simulink model "Copy_of_shunt"  (R2021a)
settings: Solver=VariableStepAuto  StartTime=0.0  StopTime=10  FixedStep=1e-6  RelTol=1e-3
libraries: spsSeriesRLCBranchLib x10, spsCurrentMeasurementLib x9, spsIGBTDiodeLib x4, spsVoltageMeasurementLib x4, spsIGBTLib x3, spsSampleandHoldLib x3, spsGroundLib x2, spsPVArrayLib x1, spsDiodeLib x1, spsPWMGeneratorDCDCLib x1, spsThreePhaseProgrammableVoltageSourceLib x1, spsUniversalBridgeLib x1
settings Model: Creator=Dell  LastModifiedBy=Dell
settings SolverCC: ZeroCrossControl=DisableAll

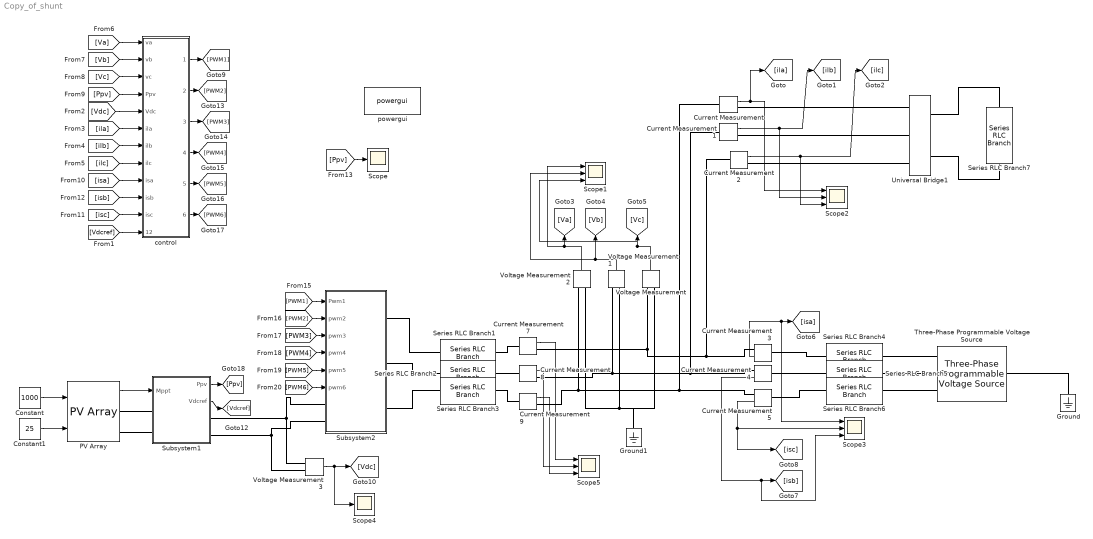
== system Copy_of_shunt ==
  Constant : Constant  Value=1000
  Constant1 : Constant  Value=25
  Current Measurement{,1..5,7..9} (9 alike) : spsCurrentMeasurementLib/Current Measurement  PhasorSimulation=off  OutputType=Complex  PSBequivalent=0
  Ground : spsGroundLib/Ground  LConnTagsString=a
  Ground1 : spsGroundLib/Ground  LConnTagsString=a
  PV Array : spsPVArrayLib/PV Array  Npar=3  Nser=25  PlotType=array @ 1000 W/m2 & specified temperatures  S_vec="[ 1000  500  100 ]"  Temp_C_vec="[ 45 25  ]"  ModuleName=User-defined  PlotWhenSelected=off  Pm=213.15  Ncell=54  Voc=36.3  Isc=7.84  Vm=29  Im=7.35  beta_Voc_pc=-0.36099  alpha_Isc_pc=0.102  beta_Voc=-0.13104  alpha_Isc=0.0079968  IL=7.8473  I0=2.9239e-10  nI=1.0901  Rsh=425.4609  Rs=0.39416  RobustModel=off  RobustCellTemperature=313.3991  BAL=on  Tc=1e-6  Tfilter=5e-5
  Scope : Scope
  Scope{1..3,5} (4 alike) : Scope  NumInputPorts=3
  Scope4 : Scope
  Series RLC Branch{1..7} (7 alike) : spsSeriesRLCBranchLib/Series RLC Branch  LConnTagsString=__new0  RConnTagsString=__new0  BranchType=RL  Resistance=1  Inductance=1e-3  SetiL0=off  InitialCurrent=0  Capacitance=1e-6  Setx0=off  InitialVoltage=0  Measurements=None
  Subsystem1 : Subsystem
  Subsystem2 : Subsystem
  Three-Phase Programmable Voltage Source : spsThreePhaseProgrammableVoltageSourceLib/Three-Phase Programmable Voltage Source  PositiveSequence="[415  0 50]"  VariationEntity=None  VariationType=Table of time-amplitude pairs  VariationTypeAlt=Step  VariationStep=0.5  VariationRate=10  VariationMagnitude=0.3  VariationFrequency=2  VariationTiming=[1 2]  VariationPhaseA=off  Amplitudes=[1 0.8 1.2 1.0]  TimeValues=[0 0.1 0.15 0.2]  HarmonicGeneration=off  HarmonicA=[3 0.2 -25 0]  HarmonicB=[2 0.15 35 2]  Timing="[0.05  3]"  BusType=swing  Pref=0  Qref=0  Qmin=-inf  Qmax=inf
  Universal Bridge1 : spsUniversalBridgeLib/Universal Bridge  Arms=3  SnubberResistance=1e5  SnubberCapacitance=inf  Device=Diodes  Ron=1e-3  Lon=0  ForwardVoltages="[  0  0  ]"  ForwardVoltage=0  GTOparameters=[ 10e-6 , 20e-6 ]  IGBTparameters=[ 1e-6 , 2e-6 ]  Measurements=None  Measurements_2=None  converterType=Rectifier
  Voltage Measurement{,1..3} (4 alike) : spsVoltageMeasurementLib/Voltage Measurement  PhasorSimulation=off  OutputType=Complex  PSBequivalent=0
  control : Subsystem
  powergui : spspowerguiLib/powergui  Priority=1  SimulationMode=Continuous  SampleTime=0.001  frequency=60  Iterations=50  frequencyindice=50  Pbase=100e6  ErrMax=1e-4  UnitsV=kV  UnitsW=MW  buscounter=0  FunctionMessages=off  echomessages=off  EnableUseOfTLC=off  CurrentSourceSwitches=off  DisableSnubberDevices=off  DisableRonSwitches=off  DisableVfSwitches=off  DisplayEquations=off  AutomaticDiscreteSolvers=off  SolverType=Tustin/Backward Euler (TBE)  Interpol=off  ExternalGateDelay=off  methode=off  Ts=100  x0status=blocks  SPID=on  SwTol=0  HookPort=off  NonlinearTolerance=1e-4  nMaxIteration=100  ContinueOnMaxIteration=off  RestoreLinks=warning  ResistiveCurrentMeasurement=off  Frange=[0:2:500]  Ylog=off  Xlog=on  ShowGrid=off  save=off  variable=ZData  structure=0  ZoomFFT=off  StartTime=0.0  cycles=1  DisplayStyle=1  fundamental=60  FreqAxis=off  MaxFrequency=1000  frequencyindicesteady=1  RmsSteady=1  display=off
  wires:
  Current Measurement/1 -> [ila], Scope2/1
  Current Measurement1/1 -> Scope2/2, [ilb]
  Current Measurement2/1 -> Scope2/3, [ilc]
  Voltage Measurement2/1 -> Scope1/1, [Va]
  Voltage Measurement1/1 -> Scope1/2, [Vb]
  Voltage Measurement/1 -> Scope1/3, [Vc]
  Current Measurement3/1 -> Scope3/1, [isa]
  Current Measurement4/1 -> Scope3/3, [isb]
  Current Measurement5/1 -> Scope3/2, [isc]
  Constant/1 -> PV Array/1
  Constant1/1 -> PV Array/2
  [Vdcref] -> control/12(Vdcref)
  [Vdc] -> control/5(Vdc)
  [ila] -> control/6(ila)
  [ilb] -> control/7(ilb)
  [ilc] -> control/8(ilc)
  [Va] -> control/1(va)
  [Vb] -> control/2(vb)
  [Vc] -> control/3(vc)
  [Ppv] -> control/4(Ppv)
  [isa] -> control/9(isa)
  [isc] -> control/11(isc)
  [isb] -> control/10(isb)
  Current Measurement7/1 -> Scope5/1
  Current Measurement8/1 -> Scope5/2
  Current Measurement9/1 -> Scope5/3
  [Ppv] -> Scope/1
  PV Array/1 -> Subsystem1/1(Mppt)
  Voltage Measurement3/1 -> Scope4/1, [Vdc]
  control/1(Output) -> [PWM1]
  control/6(Output5) -> [PWM6]
  control/5(Output4) -> [PWM5]
  control/4(Output3) -> [PWM4]
  control/3(Output2) -> [PWM3]
  control/2(Output1) -> [PWM2]
  [PWM1] -> Subsystem2/1(Pwm1)
  [PWM2] -> Subsystem2/2(pwm2)
  [PWM3] -> Subsystem2/3(pwm3)
  [PWM4] -> Subsystem2/4(pwm4)
  [PWM5] -> Subsystem2/5(pwm5)
  [PWM6] -> Subsystem2/6(pwm6)
  Subsystem1/2(Vdcref) -> [Vdcref]
  Subsystem1/1(Ppv) -> [Ppv]
  connections:
  Universal Bridge1/LConn3 -- Current Measurement/RConn1
  Universal Bridge1/LConn1 -- Current Measurement2/RConn1
  Ground/LConn1 -- Three-Phase Programmable Voltage Source/LConn1
  Current Measurement1/LConn1 -- Current Measurement8/RConn1 -- Voltage Measurement1/LConn1 -- Current Measurement4/RConn1
  Three-Phase Programmable Voltage Source/RConn1 -- Series RLC Branch4/RConn1
  Three-Phase Programmable Voltage Source/RConn2 -- Series RLC Branch5/RConn1
  Three-Phase Programmable Voltage Source/RConn3 -- Series RLC Branch6/RConn1
  Universal Bridge1/RConn1 -- Series RLC Branch7/LConn1
  Universal Bridge1/RConn2 -- Series RLC Branch7/RConn1
  Current Measurement/LConn1 -- Current Measurement9/RConn1 -- Voltage Measurement2/LConn1 -- Current Measurement5/RConn1
  Universal Bridge1/LConn2 -- Current Measurement1/RConn1
  Current Measurement2/LConn1 -- Voltage Measurement/LConn1 -- Current Measurement7/RConn1 -- Current Measurement3/RConn1
  Voltage Measurement2/LConn2 -- Voltage Measurement/LConn2 -- Ground1/LConn1 -- Voltage Measurement1/LConn2
  Series RLC Branch4/LConn1 -- Current Measurement3/LConn1
  Series RLC Branch5/LConn1 -- Current Measurement4/LConn1
  Series RLC Branch6/LConn1 -- Current Measurement5/LConn1
  Current Measurement7/LConn1 -- Series RLC Branch1/RConn1
  Current Measurement8/LConn1 -- Series RLC Branch2/RConn1
  Current Measurement9/LConn1 -- Series RLC Branch3/RConn1
  Subsystem1/LConn1 -- PV Array/RConn1
  Subsystem1/LConn2 -- PV Array/RConn2
  Subsystem1/RConn1 -- Voltage Measurement3/LConn1 -- Subsystem2/LConn1
  Subsystem1/RConn2 -- Voltage Measurement3/LConn2 -- Subsystem2/LConn2
  Series RLC Branch1/LConn1 -- Subsystem2/RConn1
  Series RLC Branch2/LConn1 -- Subsystem2/RConn2
  Series RLC Branch3/LConn1 -- Subsystem2/RConn3

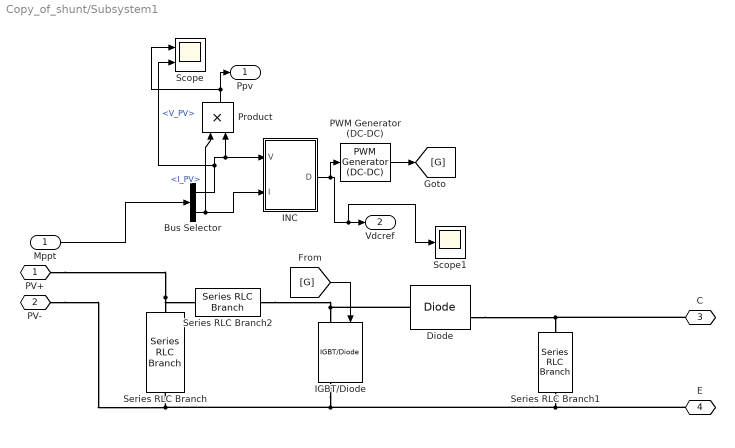
== system Copy_of_shunt/Subsystem1 ==
  Mppt : Inport
  Bus Selector : BusSelector  OutputSignals=V_PV,I_PV
  Diode : spsDiodeLib/Diode  Ron=0.001  Lon=0  Vf=0.8  IC=0  UseSnubber=0  Rs=500  Cs=250e-9  Measurements=on
  IGBT/Diode : spsIGBTDiodeLib/IGBT//Diode  Ron=1e-3  Rs=1e5  Cs=inf  Measurements=on
  INC : Subsystem
  PWM Generator (DC-DC) : spsPWMGeneratorDCDCLib/PWM Generator (DC-DC)  Fsw=5000  Ts=0
  Product : Product
  Scope : Scope  NumInputPorts=2
  Scope1 : Scope
  Series RLC Branch : spsSeriesRLCBranchLib/Series RLC Branch  LConnTagsString=__new0  RConnTagsString=__new0  BranchType=RC  Resistance=1  Inductance=1e-3  SetiL0=off  InitialCurrent=0  Capacitance=1e-6  Setx0=off  InitialVoltage=0  Measurements=None
  Series RLC Branch1 : spsSeriesRLCBranchLib/Series RLC Branch  LConnTagsString=__new0  RConnTagsString=__new0  BranchType=C  Resistance=1  Inductance=1e-3  SetiL0=off  InitialCurrent=0  Capacitance=1e-6  Setx0=off  InitialVoltage=0  Measurements=None
  Series RLC Branch2 : spsSeriesRLCBranchLib/Series RLC Branch  LConnTagsString=__new0  RConnTagsString=__new0  BranchType=L  Resistance=1  Inductance=1e-3  SetiL0=off  InitialCurrent=0  Capacitance=1e-6  Setx0=off  InitialVoltage=0  Measurements=None
  PV+ : PMIOPort  Side=Left
  PV- : PMIOPort  Port=2  Side=Left
  C : PMIOPort  Port=3  Side=Right
  E : PMIOPort  Port=4  Side=Right
  Ppv : Outport
  Vdcref : Outport  Port=2
  wires:
  INC/1(D) -> PWM Generator (DC-DC)/1, Scope1/1, Vdcref/1
  Bus Selector/2 -> INC/2(I), Product/1  "<I_PV>"
  Bus Selector/1 -> Scope/2, Product/2, INC/1(V)  "<V_PV>"
  [G] -> IGBT/Diode/1
  PWM Generator (DC-DC)/1 -> [G]
  Mppt/1 -> Bus Selector/1
  Product/1 -> Scope/1, Ppv/1
  connections:
  IGBT/Diode/RConn1 -- E/RConn1 -- Series RLC Branch1/RConn1 -- PV-/RConn1 -- Series RLC Branch/RConn1
  Diode/RConn1 -- C/RConn1 -- Series RLC Branch1/LConn1
  IGBT/Diode/LConn1 -- Series RLC Branch2/RConn1 -- Diode/LConn1
  Series RLC Branch/LConn1 -- PV+/RConn1 -- Series RLC Branch2/LConn1

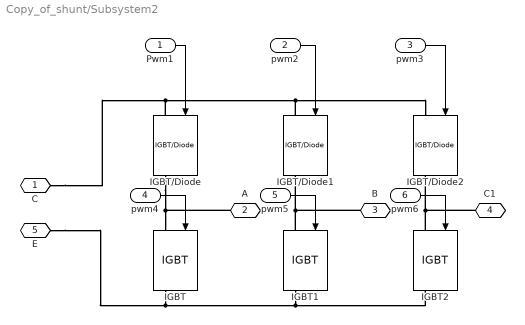
== system Copy_of_shunt/Subsystem2 ==
  Pwm1 : Inport
  pwm2 : Inport  Port=2
  pwm3 : Inport  Port=3
  pwm4 : Inport  Port=4
  pwm5 : Inport  Port=5
  pwm6 : Inport  Port=6
  IGBT : spsIGBTLib/IGBT  Ron=0.001  Lon=0  Vf=1  Tf=1e-6  Tt=2e-6  IC=0  Rs=1e5  Cs=inf  Measurements=on
  IGBT/Diode : spsIGBTDiodeLib/IGBT//Diode  Ron=1e-3  Rs=1e5  Cs=inf  Measurements=on
  IGBT/Diode1 : spsIGBTDiodeLib/IGBT//Diode  Ron=1e-3  Rs=1e5  Cs=inf  Measurements=on
  IGBT/Diode2 : spsIGBTDiodeLib/IGBT//Diode  Ron=1e-3  Rs=1e5  Cs=inf  Measurements=on
  IGBT1 : spsIGBTLib/IGBT  Ron=0.001  Lon=0  Vf=1  Tf=1e-6  Tt=2e-6  IC=0  Rs=1e5  Cs=inf  Measurements=on
  IGBT2 : spsIGBTLib/IGBT  Ron=0.001  Lon=0  Vf=1  Tf=1e-6  Tt=2e-6  IC=0  Rs=1e5  Cs=inf  Measurements=on
  C : PMIOPort  Side=Left
  A : PMIOPort  Port=2  Side=Right
  B : PMIOPort  Port=3  Side=Right
  C1 : PMIOPort  Port=4  Side=Right
  E : PMIOPort  Port=5  Side=Left
  wires:
  Pwm1/1 -> IGBT/Diode/1
  pwm6/1 -> IGBT2/1
  pwm5/1 -> IGBT1/1
  pwm4/1 -> IGBT/1
  pwm3/1 -> IGBT/Diode2/1
  pwm2/1 -> IGBT/Diode1/1
  connections:
  IGBT/Diode/RConn1 -- A/RConn1 -- IGBT/LConn1
  IGBT1/LConn1 -- B/RConn1 -- IGBT/Diode1/RConn1
  IGBT2/LConn1 -- C1/RConn1 -- IGBT/Diode2/RConn1
  IGBT/Diode/LConn1 -- C/RConn1 -- IGBT/Diode1/LConn1 -- IGBT/Diode2/LConn1
  IGBT/RConn1 -- E/RConn1 -- IGBT1/RConn1 -- IGBT2/RConn1

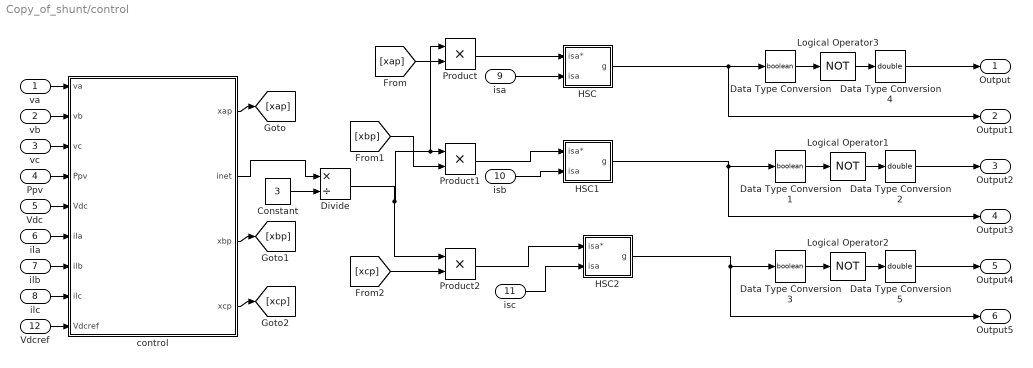
== system Copy_of_shunt/control ==
  va : Inport
  vb : Inport  Port=2
  vc : Inport  Port=3
  Ppv : Inport  Port=4
  Vdc : Inport  Port=5
  ila : Inport  Port=6
  ilb : Inport  Port=7
  ilc : Inport  Port=8
  isa : Inport  Port=9
  isb : Inport  Port=10
  isc : Inport  Port=11
  Vdcref : Inport  Port=12
  Constant : Constant  Value=3
  Data Type Conversion : DataTypeConversion  OutDataTypeStr=boolean  SaturateOnIntegerOverflow=on  RndMeth=Zero
  Data Type Conversion1 : DataTypeConversion  OutDataTypeStr=boolean  SaturateOnIntegerOverflow=on  RndMeth=Zero
  Data Type Conversion2 : DataTypeConversion  OutDataTypeStr=double  SaturateOnIntegerOverflow=on  RndMeth=Zero
  Data Type Conversion3 : DataTypeConversion  OutDataTypeStr=boolean  SaturateOnIntegerOverflow=on  RndMeth=Zero
  Data Type Conversion4 : DataTypeConversion  OutDataTypeStr=double  SaturateOnIntegerOverflow=on  RndMeth=Zero
  Data Type Conversion5 : DataTypeConversion  OutDataTypeStr=double  SaturateOnIntegerOverflow=on  RndMeth=Zero
  Divide : Product  Inputs=*/
  HSC : Subsystem  mask{h=.1}
      mask prompts: h "Hysteresis band (A)"
      mask help: Hysteresis Current Controller
      mask Display: plot(0,0,100,100,[45,45],[35,65],[55,55],[35,65],[45,65],[65,65],[35,55],[35,35])
  HSC1 : Subsystem  mask{h=.1}
      mask prompts: h "Hysteresis band (A)"
      mask help: Hysteresis Current Controller
      mask Display: plot(0,0,100,100,[45,45],[35,65],[55,55],[35,65],[45,65],[65,65],[35,55],[35,35])
  HSC2 : Subsystem  mask{h=.1}
      mask prompts: h "Hysteresis band (A)"
      mask help: Hysteresis Current Controller
      mask Display: plot(0,0,100,100,[45,45],[35,65],[55,55],[35,65],[45,65],[65,65],[35,55],[35,35])
  Logical Operator1 : Logic  Operator=NOT  AllPortsSameDT=off  OutDataTypeStr=boolean
  Logical Operator2 : Logic  Operator=NOT  AllPortsSameDT=off  OutDataTypeStr=boolean
  Logical Operator3 : Logic  Operator=NOT  AllPortsSameDT=off  OutDataTypeStr=boolean
  Product : Product
  Product1 : Product
  Product2 : Product
  control : Subsystem
  Output : Outport
  Output1 : Outport  Port=2
  Output2 : Outport  Port=3
  Output3 : Outport  Port=4
  Output4 : Outport  Port=5
  Output5 : Outport  Port=6
  wires:
  Product/1 -> HSC/1(isa*)
  Constant/1 -> Divide/2
  Divide/1 -> Product2/1, Product1/1, Product/1
  Product2/1 -> HSC2/1(isa*)
  [xcp] -> Product2/2
  isa/1 -> HSC/2(isa)
  Product1/1 -> HSC1/1(isa*)
  [xbp] -> Product1/2
  control/2(inet) -> Divide/1
  Logical Operator1/1 -> Data Type Conversion2/1
  HSC2/1(g) -> Output5/1, Data Type Conversion3/1
  Data Type Conversion4/1 -> Output/1
  HSC1/1(g) -> Output3/1, Data Type Conversion1/1
  Data Type Conversion1/1 -> Logical Operator1/1
  Data Type Conversion5/1 -> Output4/1
  Data Type Conversion3/1 -> Logical Operator2/1
  HSC/1(g) -> Output1/1, Data Type Conversion/1
  Data Type Conversion/1 -> Logical Operator3/1
  Data Type Conversion2/1 -> Output2/1
  Logical Operator2/1 -> Data Type Conversion5/1
  Logical Operator3/1 -> Data Type Conversion4/1
  control/1(xap) -> [xap]
  [xap] -> Product/2
  control/3(xbp) -> [xbp]
  control/4(xcp) -> [xcp]
  va/1 -> control/1(va)
  vb/1 -> control/2(vb)
  vc/1 -> control/3(vc)
  Ppv/1 -> control/4(Ppv)
  Vdc/1 -> control/5(Vdc)
  ila/1 -> control/6(ila)
  ilb/1 -> control/7(ilb)
  ilc/1 -> control/8(ilc)
  isb/1 -> HSC1/2(isa)
  isc/1 -> HSC2/2(isa)
  Vdcref/1 -> control/9(Vdcref)

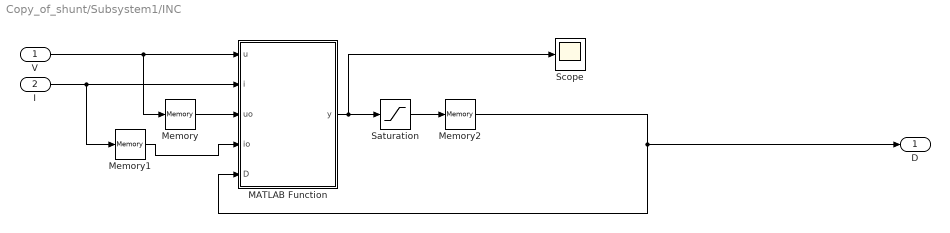
== system Copy_of_shunt/Subsystem1/INC ==
  V : Inport
  I : Inport  Port=2
  MATLAB Function : MATLAB Function  TreatAsAtomicUnit=on
  Memory : Memory  InheritSampleTime=on
  Memory1 : Memory  InheritSampleTime=on
  Memory2 : Memory  InheritSampleTime=on
  Saturation : Saturate  UpperLimit=0.9  LowerLimit=0
  Scope : Scope
  D : Outport
  wires:
  Memory/1 -> MATLAB Function/3(uo)
  Saturation/1 -> Memory2/1
  V/1 -> Memory/1, MATLAB Function/1(u)
  Memory1/1 -> MATLAB Function/4(io)
  I/1 -> Memory1/1, MATLAB Function/2(i)
  Memory2/1 -> D/1, MATLAB Function/5(D)
  MATLAB Function/1(y) -> Scope/1, Saturation/1

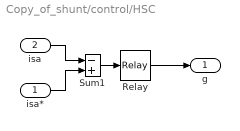
== system Copy_of_shunt/control/HSC ==
  isa* : Inport
  isa : Inport  Port=2
  Relay : Relay  OnSwitchValue=h/2  OffSwitchValue=-h/2  ZeroCross=off
  Sum1 : Sum  Inputs=-+  InputSameDT=on  SaturateOnIntegerOverflow=on  OutDataTypeStr=Inherit: Same as first input
  g : Outport  InitialOutput=0
  wires:
  Sum1/1 -> Relay/1
  Relay/1 -> g/1
  isa/1 -> Sum1/1
  isa*/1 -> Sum1/2

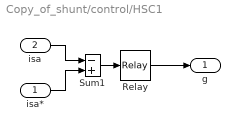
== system Copy_of_shunt/control/HSC1 ==
  isa* : Inport
  isa : Inport  Port=2
  Relay : Relay  OnSwitchValue=h/2  OffSwitchValue=-h/2
  Sum1 : Sum  Inputs=-+  InputSameDT=on  SaturateOnIntegerOverflow=on  OutDataTypeStr=Inherit: Same as first input
  g : Outport  InitialOutput=0
  wires:
  Sum1/1 -> Relay/1
  Relay/1 -> g/1
  isa/1 -> Sum1/1
  isa*/1 -> Sum1/2

== system Copy_of_shunt/control/HSC2 ==
  isa* : Inport
  isa : Inport  Port=2
  Relay : Relay  OnSwitchValue=h/2  OffSwitchValue=-h/2
  Sum1 : Sum  Inputs=-+  InputSameDT=on  SaturateOnIntegerOverflow=on  OutDataTypeStr=Inherit: Same as first input
  g : Outport  InitialOutput=0
  wires:
  Sum1/1 -> Relay/1
  Relay/1 -> g/1
  isa/1 -> Sum1/1
  isa*/1 -> Sum1/2

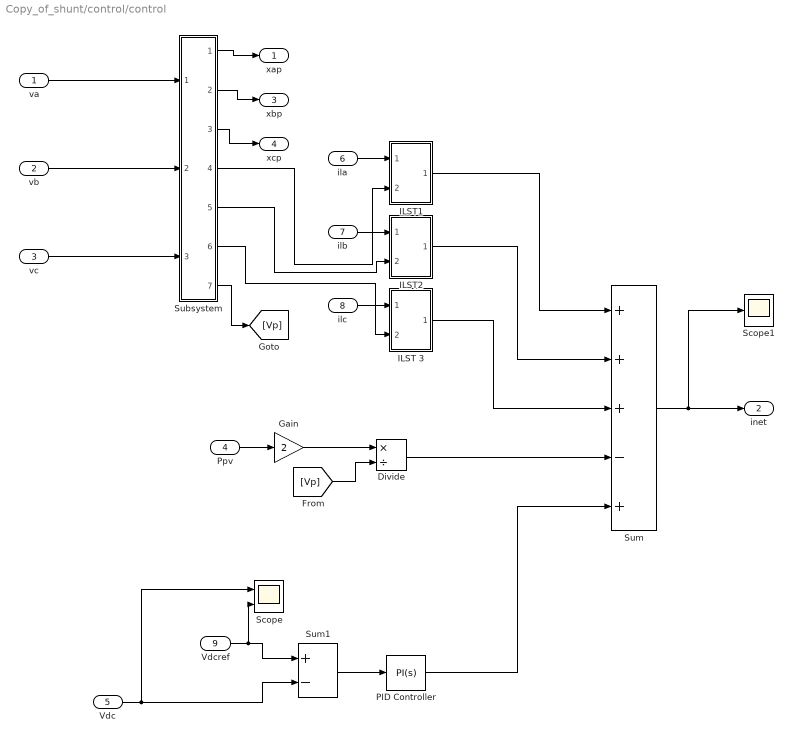
== system Copy_of_shunt/control/control ==
  va : Inport
  vb : Inport  Port=2
  vc : Inport  Port=3
  Ppv : Inport  Port=4
  Vdc : Inport  Port=5
  ila : Inport  Port=6
  ilb : Inport  Port=7
  ilc : Inport  Port=8
  Vdcref : Inport  Port=9
  Divide : Product  Inputs=*/
  Gain : Gain  Gain=2
  ILST 3 : Subsystem
  ILST1 : Subsystem
  ILST2 : Subsystem
  PID Controller : pid_lib/PID Controller  Controller=PI  Form=Parallel  TimeDomain=Continuous-time  UseExternalTs=off  SampleTime=-1  IntegratorMethod=Forward Euler  FilterMethod=Forward Euler  ControllerParametersSource=internal  P=1  I=1  D=0  UseFilter=on  N=100  TunerSelectOption=Transfer Function Based (PID Tuner App)  InitialConditionSource=internal  InitialConditionForIntegrator=0  InitialConditionForFilter=0  DifferentiatorICPrevScaledInput=0  ExternalReset=none  TrackingMode=off  Kt=1  LimitOutput=off  SatLimitsSource=internal  UpperSaturationLimit=inf  LowerSaturationLimit=-inf  LinearizeAsGain=on  AntiWindupMode=none  Kb=1  POutMin=[]  POutMax=[]  IOutMin=[]  IOutMax=[]  DOutMin=[]  DOutMax=[]  NOutMin=[]  NOutMax=[]  SumOutMin=[]  SumOutMax=[]  SaturationOutMin=[]  SaturationOutMax=[]  PParamMin=[]  PParamMax=[]  IParamMin=[]  IParamMax=[]  DParamMin=[]  DParamMax=[]  NParamMin=[]  NParamMax=[]  KbParamMin=[]  KbParamMax=[]  KtParamMin=[]  KtParamMax=[]  KbOutMin=[]  KbOutMax=[]  KtOutMin=[]  KtOutMax=[]  IntegratorOutMin=[]  IntegratorOutMax=[]  FilterOutMin=[]  FilterOutMax=[]  SumI1OutMin=[]  SumI1OutMax=[]  SumI2OutMin=[]  SumI2OutMax=[]  SumI3OutMin=[]  SumI3OutMax=[]  SumI4OutMin=[]  SumI4OutMax=[]  SumDOutMin=[]  SumDOutMax=[]  DifferentiatorOutMin=[]  DifferentiatorOutMax=[]  FilterDiffOutCoefMin=[]  FilterDiffOutCoefMax=[]  ReciprocalOutMin=[]  ReciprocalOutMax=[]  SumDenOutMin=[]  SumDenOutMax=[]  SumNumOutMin=[]  SumNumOutMax=[]  DivideOutMin=[]  DivideOutMax=[]  UdiffTsProdOutMin=[]  UdiffTsProdOutMax=[]  NTsProdOutMin=[]  NTsProdOutMax=[]  UintegralTsProdOutMin=[]  UintegralTsProdOutMax=[]  UngainTsProdOutMin=[]  UngainTsProdOutMax=[]  IntegratorContinuousStateAttributes=''  IntegratorStateMustResolveToSignalObject=off  IntegratorRTWStateStorageClass=Auto  FilterContinuousStateAttributes=''  FilterStateMustResolveToSignalObject=off  FilterRTWStateStorageClass=Auto  ParallelPVariant=InternalParameters  IdealPVariant=Disabled  IVariant=InternalParameters  DVariant=Disabled  IntegratorVariant=Continuous  SatVariant=Disabled  AWVariant=Passthrough  PCopyVariant=Disabled  TRVariant=Disabled  FdbkBlocksVariant=Forward  IdealPFdbkVariant=Disabled  SatFdbkVariant=Disabled  DerivativeFilterVariant=Disabled  NVariant=Disabled  NCopyVariant=Disabled_SignalSpec  FilterICVariant=Disabled  IntegratorICVariant=InternalICs  ExternalResetVariant=Disabled  TRSumVariant=Passthrough  SumFdbkVariant=Disabled  SumVariant=Sum_PI  TsampFilterVariant=InternalTs  TsampNgainVariant=Passthrough  TsampIntegralVariant=Passthrough  ExternalSaturationOutDataTypeStr=Inherit: Same as second input
  Scope : Scope  NumInputPorts=2
  Scope1 : Scope
  Subsystem : Subsystem
  Sum : Sum  Inputs=+++-+
  Sum1 : Sum  Inputs=+-
  xap : Outport
  inet : Outport  Port=2
  xbp : Outport  Port=3
  xcp : Outport  Port=4
  wires:
  Vdcref/1 -> Scope/2, Sum1/1
  ILST2/1(Out1) -> Sum/2
  Sum1/1 -> PID Controller/1
  Ppv/1 -> Gain/1
  ILST1/1(Out1) -> Sum/1
  ILST 3/1(Out1) -> Sum/3
  Vdc/1 -> Sum1/2, Scope/1
  Divide/1 -> Sum/4
  PID Controller/1 -> Sum/5
  Gain/1 -> Divide/1
  Sum/1 -> Scope1/1, inet/1
  vc/1 -> Subsystem/3(Input2)
  vb/1 -> Subsystem/2(Input1)
  va/1 -> Subsystem/1(Input)
  ila/1 -> ILST1/1(In1)
  Subsystem/2(Out2) -> xbp/1
  Subsystem/1(Out1) -> xap/1
  ilb/1 -> ILST2/1(In1)
  Subsystem/6(Out6) -> ILST 3/2(In2)
  Subsystem/5(Out5) -> ILST2/2(In2)
  ilc/1 -> ILST 3/1(In1)
  Subsystem/3(Out3) -> xcp/1
  Subsystem/4(Out4) -> ILST1/2(In2)
  Subsystem/7(Vp) -> [Vp]
  [Vp] -> Divide/2

== system Copy_of_shunt/control/control/ILST 3 ==
  In1 : Inport
  In2 : Inport  Port=2
  ILST3 : Subsystem
  Out1 : Outport
  wires:
  In1/1 -> ILST3/1(In1)
  In2/1 -> ILST3/2(In2)
  ILST3/1(Out1) -> Out1/1

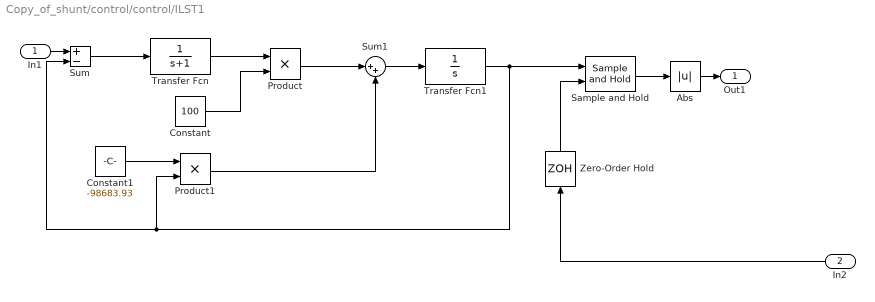
== system Copy_of_shunt/control/control/ILST1 ==
  In1 : Inport
  In2 : Inport  Port=2
  Abs : Abs  ZeroCross=off
  Constant : Constant  Value=100
  Constant1 : Constant  Value=-98683.93
  Product : Product
  Product1 : Product
  Sample and Hold : spsSampleandHoldLib/Sample and Hold  ic=0  Ts=0
      settings: SourceProductBaseCode=PS
  Sum : Sum  Inputs=+-
  Sum1 : Sum  Inputs=|++
  Transfer Fcn : TransferFcn  Denominator=[1 1]
  Transfer Fcn1 : TransferFcn  Denominator=[1 0]
  Zero-Order Hold : ZeroOrderHold  SampleTime=-1
  Out1 : Outport
  wires:
  Constant/1 -> Product/2
  Constant1/1 -> Product1/1
  Product/1 -> Sum1/1
  Zero-Order Hold/1 -> Sample and Hold/2
  Sum1/1 -> Transfer Fcn1/1
  In1/1 -> Sum/1
  Transfer Fcn1/1 -> Sample and Hold/1, Product1/2, Sum/2
  Product1/1 -> Sum1/2
  Transfer Fcn/1 -> Product/1
  Sum/1 -> Transfer Fcn/1
  Sample and Hold/1 -> Abs/1
  In2/1 -> Zero-Order Hold/1
  Abs/1 -> Out1/1

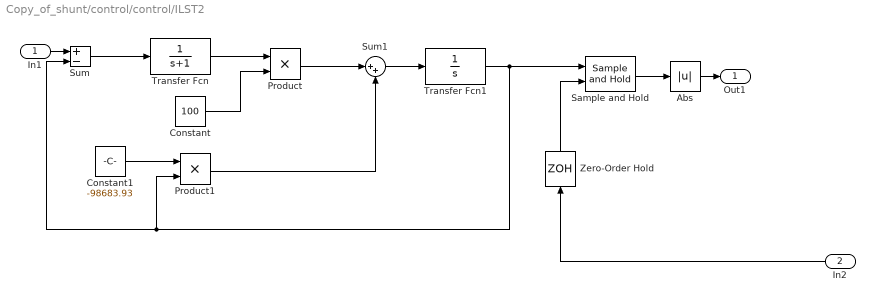
== system Copy_of_shunt/control/control/ILST2 ==
  In1 : Inport
  In2 : Inport  Port=2
  Abs : Abs  ZeroCross=off
  Constant : Constant  Value=100
  Constant1 : Constant  Value=-98683.93
  Product : Product
  Product1 : Product
  Sample and Hold : spsSampleandHoldLib/Sample and Hold  ic=0  Ts=0
      settings: SourceProductBaseCode=PS
  Sum : Sum  Inputs=+-
  Sum1 : Sum  Inputs=|++
  Transfer Fcn : TransferFcn  Denominator=[1 1]
  Transfer Fcn1 : TransferFcn  Denominator=[1 0]
  Zero-Order Hold : ZeroOrderHold  SampleTime=-1
  Out1 : Outport
  wires:
  Constant/1 -> Product/2
  Constant1/1 -> Product1/1
  Product/1 -> Sum1/1
  Zero-Order Hold/1 -> Sample and Hold/2
  Sum1/1 -> Transfer Fcn1/1
  In1/1 -> Sum/1
  Transfer Fcn1/1 -> Sample and Hold/1, Product1/2, Sum/2
  Product1/1 -> Sum1/2
  Transfer Fcn/1 -> Product/1
  Sum/1 -> Transfer Fcn/1
  Sample and Hold/1 -> Abs/1
  In2/1 -> Zero-Order Hold/1
  Abs/1 -> Out1/1

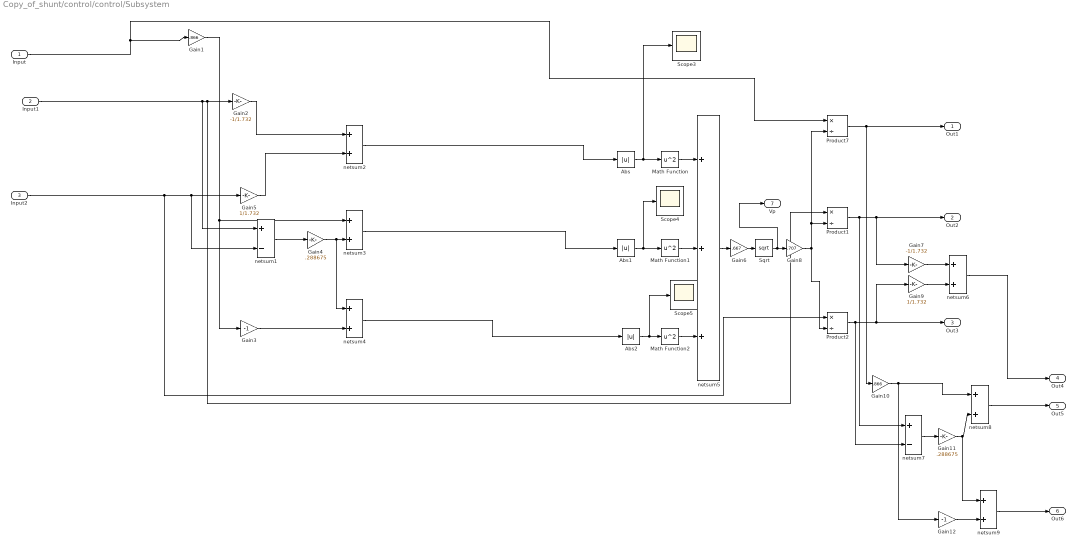
== system Copy_of_shunt/control/control/Subsystem ==
  Input : Inport
  Input1 : Inport  Port=2
  Input2 : Inport  Port=3
  Abs : Abs
  Abs1 : Abs
  Abs2 : Abs
  Gain1 : Gain  Gain=.866
  Gain10 : Gain  Gain=.866
  Gain11 : Gain  Gain=.288675
  Gain12 : Gain  Gain=-1
  Gain2 : Gain  Gain=-1/1.732
  Gain3 : Gain  Gain=-1
  Gain4 : Gain  Gain=.288675
  Gain5 : Gain  Gain=1/1.732
  Gain6 : Gain  Gain=.667
  Gain7 : Gain  Gain=-1/1.732
  Gain8 : Gain  Gain=.707
  Gain9 : Gain  Gain=1/1.732
  Math Function : Math  Operator=square  SignedPower=on  SaturateOnIntegerOverflow=on
  Math Function1 : Math  Operator=square  SignedPower=on  SaturateOnIntegerOverflow=on
  Math Function2 : Math  Operator=square  SignedPower=on  SaturateOnIntegerOverflow=on
  Product1 : Product  Inputs=*/  RndMeth=Zero
  Product2 : Product  Inputs=*/  RndMeth=Zero
  Product7 : Product  Inputs=*/  RndMeth=Zero
  Scope3 : Scope
  Scope4 : Scope
  Scope5 : Scope
  Sqrt : Sqrt  SaturateOnIntegerOverflow=on
  netsum1 : Sum  Inputs=+-  InputSameDT=on  SaturateOnIntegerOverflow=on  OutDataTypeStr=Inherit: Same as first input
  netsum{2..4,6,8..9} (6 alike) : Sum  InputSameDT=on  SaturateOnIntegerOverflow=on  OutDataTypeStr=Inherit: Same as first input
  netsum5 : Sum  Inputs=+++  InputSameDT=on  SaturateOnIntegerOverflow=on  OutDataTypeStr=Inherit: Same as first input
  netsum7 : Sum  Inputs=+-  InputSameDT=on  SaturateOnIntegerOverflow=on  OutDataTypeStr=Inherit: Same as first input
  Out1 : Outport
  Out2 : Outport  Port=2
  Out3 : Outport  Port=3
  Out4 : Outport  Port=4
  Out5 : Outport  Port=5
  Out6 : Outport  Port=6
  Vp : Outport  Port=7
  wires:
  Input2/1 -> Product2/1, netsum1/2, Gain5/1
  Input1/1 -> netsum1/1, Product1/1, Gain2/1
  Gain9/1 -> netsum6/2
  Gain8/1 -> Product2/2, Product7/2, Product1/2
  Gain12/1 -> netsum9/2
  netsum2/1 -> Abs/1
  netsum9/1 -> Out6/1
  Gain3/1 -> netsum4/2
  netsum7/1 -> Gain11/1
  Gain4/1 -> netsum4/1, netsum3/2
  Gain5/1 -> netsum2/2
  netsum1/1 -> Gain4/1
  Math Function2/1 -> netsum5/3
  Gain1/1 -> Gain3/1, netsum3/1
  netsum8/1 -> Out5/1
  Product7/1 -> Gain10/1, Out1/1
  Gain2/1 -> netsum2/1
  Product2/1 -> netsum7/2, Gain9/1, Out3/1
  Math Function/1 -> netsum5/1
  Input/1 -> Product7/1, Gain1/1
  Product1/1 -> netsum7/1, Out2/1, Gain7/1
  netsum3/1 -> Abs1/1
  Sqrt/1 -> Vp/1, Gain8/1
  Abs2/1 -> Scope5/1, Math Function2/1
  Gain11/1 -> netsum9/1, netsum8/2
  Abs1/1 -> Scope4/1, Math Function1/1
  netsum5/1 -> Gain6/1
  Gain6/1 -> Sqrt/1
  Math Function1/1 -> netsum5/2
  netsum4/1 -> Abs2/1
  Gain7/1 -> netsum6/1
  netsum6/1 -> Out4/1
  Gain10/1 -> Gain12/1, netsum8/1
  Abs/1 -> Scope3/1, Math Function/1

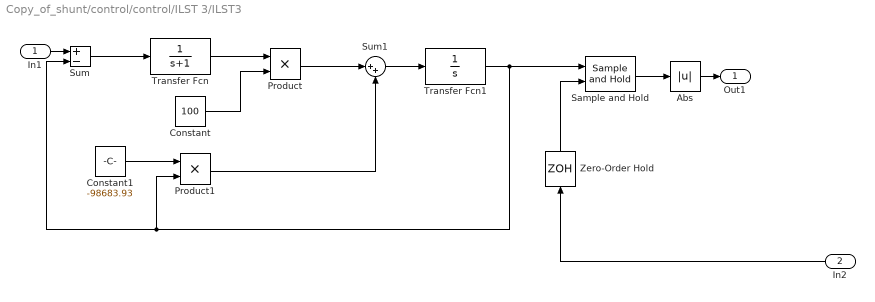
== system Copy_of_shunt/control/control/ILST 3/ILST3 ==
  In1 : Inport
  In2 : Inport  Port=2
  Abs : Abs  ZeroCross=off
  Constant : Constant  Value=100
  Constant1 : Constant  Value=-98683.93
  Product : Product
  Product1 : Product
  Sample and Hold : spsSampleandHoldLib/Sample and Hold  ic=0  Ts=0
      settings: SourceProductBaseCode=PS
  Sum : Sum  Inputs=+-
  Sum1 : Sum  Inputs=|++
  Transfer Fcn : TransferFcn  Denominator=[1 1]
  Transfer Fcn1 : TransferFcn  Denominator=[1 0]
  Zero-Order Hold : ZeroOrderHold  SampleTime=-1
  Out1 : Outport
  wires:
  Constant/1 -> Product/2
  Constant1/1 -> Product1/1
  Product/1 -> Sum1/1
  Zero-Order Hold/1 -> Sample and Hold/2
  Sum1/1 -> Transfer Fcn1/1
  In1/1 -> Sum/1
  Transfer Fcn1/1 -> Sample and Hold/1, Product1/2, Sum/2
  Product1/1 -> Sum1/2
  Transfer Fcn/1 -> Product/1
  Sum/1 -> Transfer Fcn/1
  Sample and Hold/1 -> Abs/1
  In2/1 -> Zero-Order Hold/1
  Abs/1 -> Out1/1

== matlab function Copy_of_shunt/Subsystem1/INC/MATLAB Function ==
  data: u input; y output; i input; uo input; io input; D input
function y = MYMPP(u,i,uo,io,D)
m=0.4;
du=u-uo;
di=i-io;
d=0.00005;
if du==0
    if di==0
    m=D;
    else
        if di>0
            m=D-d;
        else
            m=D+d;
        end
    end
else
    if di/du== -(i/u)
    m=D;
    else
        if di/du> -(i/u)
        m=D-d;
        else
            m=D+d;
        end
    end
end
y = m;
end
